simulink model "f"  (R2019a)
settings: Solver=VariableStepAuto  StartTime=0.0  StopTime=10.0  RelTol=1e-3
settings Model: Creator=nfoin  LastModifiedBy=nfoin

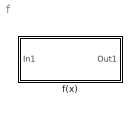
== system f ==
  f(x) : Subsystem

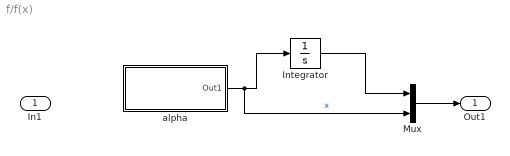
== system f/f(x) ==
  In1 : Inport
  Integrator : Integrator
  Mux : Mux  Inputs=2
  alpha : Subsystem
  Out1 : Outport
  wires:
  alpha/1(Out1) -> Mux/2, Integrator/1  "x"
  Integrator/1 -> Mux/1
  Mux/1 -> Out1/1

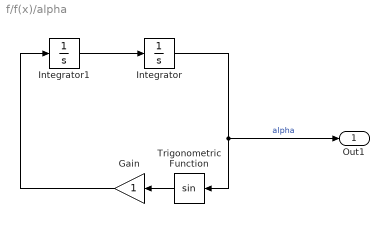
== system f/f(x)/alpha ==
  Gain : Gain
  Integrator : Integrator
  Integrator1 : Integrator  InitialCondition=1
  Trigonometric Function : Trigonometry
  Out1 : Outport
  wires:
  Gain/1 -> Integrator1/1
  Trigonometric Function/1 -> Gain/1
  Integrator/1 -> Out1/1, Trigonometric Function/1  "alpha"
  Integrator1/1 -> Integrator/1
